simulink model "LGS_allFaultsDeselected"  (R2019b)
settings: Solver=FixedStepDiscrete  StartTime=0.0  StopTime=45.0  FixedStep=0.1  RelTol=1e-3
model workspace (MAT data in the model file):
  fipData : object (value not decoded)
  fipName : object (value not decoded)
  stepSize = 0.1
libraries: LibFaultInjectionControls x190, commrandsrc3 x70, simulink x3, LibFailureCondition x1
(part 3 of 41)

== system LGS_allFaultsDeselected/Doors/EV open doors ==
  In1 : Inport
  In2 : Inport  Port=2
  EV open doors : Stateflow chart  TreatAsAtomicUnit=on
  EV open doors FIP : Subsystem  Commented=on  mask(FailureInjectionPoint){}
      mask help: FailureInjectionPoint
      mask init: same as LGS_allFaultsDeselected/Analogical switch and general electro-valve and pressure sensor/Analogical switch/Analog Switch FIP
      settings: OpenFcn=|
      | open_system(gcb,'mask');
      | 
      | treeValues = FailureInjectionPointHelper.getAllFmAndParamsAsTreeString(gcb);
      | mo = Simulink.Mask.get(gcb);
      | dc = mo.getDialogControl('GbFmInfo');
      | treeView = dc.getDialogControl('TreeViewFM');
      | treeView.TreeItems = {};
      | treeView.TreeItems = treeValues;
      mask Help: FailureInjectionPoint
      mask DialogControl Control7 Prompt: Containing Failure Modes
      mask DialogControl BtnMoveUp Prompt: Move up
      mask DialogControl BtnMoveUp Callback:
      | %Get name of the failure mode block
      | mo = Simulink.Mask.get(gcb);
      | dc = mo.getDialogControl('GbFmInfo');
      | treeView = dc.getDialogControl('TreeViewFM');
      | try
      |     a = treeView.getSelectedItems();
      |     p = split(a, '/'); %name of failure mode block is p{1}
      | catch
      |     return;
      | end
      | 
      | %Save port handles
      | lh = get_param([gcb,'/',p{1}],'LineHandles');
      | ph = get_param([gcb,'/',p{1}],'PortHandles');
      | this_in = ph.Inport(1);
      | this_out = ph.Outport(1);
      | 
      | last_block = get_param(lh.Inport(1),'SrcBlockHandle');
      | last_block_type = get_param(last_block,'BlockType');
      | if strcmp(last_block_type,'Inport')
      |     return;
      | end
      | lb_lh = get_param(last_block,'LineHandles');
      | 
      | last_out = get_param(lh.Inport(1),'SrcPortHandle');
      | last_in = get_param(lb_lh.Inport(1),'DstPortHandle');
      | next_to_last_out = get_param(lb_lh.Inport(1),'SrcPortHandle');
      | next_in = get_param(lh.Outport(1),'DstPortHandle');
      | 
      | %Delete connecting lines
      | delete_line(lh.Inport(1));
      | delete_line(lh.Outport(1));
      | delete_line(lb_lh.Inport(1));
      | 
      | % Generate new lines
      | add_line(gcb, last_out, next_in, 'autorouting', 'smart');
      | add_line(gcb, this_out, last_in, 'autorouting', 'smart');
      | add_line(gcb, next_to_last_out, this_in, 'autorouting', 'smart');
      | 
      | %Rearrange system
      | Simulink.BlockDiagram.arrangeSystem(gcb);
      | 
      | %Refresh
      | treeValues = FailureInjectionPointHelper.getAllFmAndParamsAsTreeString(gcb);
      | mo = Simulink.Mask.get(gcb);
      | dc = mo.getDialogControl('GbFmInfo');
      | treeView = dc.getDialogControl('TreeViewFM');
      | treeView.TreeItems = {};
      | treeView.TreeItems = treeValues;
      mask DialogControl BtnMoveDown Prompt: Move down
      mask DialogControl BtnMoveDown Callback:
      | %Get name of the failure mode block
      | mo = Simulink.Mask.get(gcb);
      | dc = mo.getDialogControl('GbFmInfo');
      | treeView = dc.getDialogControl('TreeViewFM');
      | try
      |     a = treeView.getSelectedItems();
      |     p = split(a, '/'); %name of failure mode block is p{1}
      | catch
      |     return;
      | end
      | 
      | %Save port handles
      | lh = get_param([gcb,'/',p{1}],'LineHandles');
      | ph = get_param([gcb,'/',p{1}],'PortHandles');
      | this_in = ph.Inport(1);
      | this_out = ph.Outport(1);
      | 
      | next_block = get_param(lh.Outport(1),'DstBlockHandle');
      | next_block_type = get_param(next_block,'BlockType');
      | if strcmp(next_block_type,'Outport')
      |     return;
      | end
      | nb_lh = get_param(next_block,'LineHandles');
      | 
      | last_out = get_param(lh.Inport(1),'SrcPortHandle');
      | next_out = get_param(nb_lh.Outport(1),'SrcPortHandle');
      | next_but_one_in = get_param(nb_lh.Outport(1),'DstPortHandle');
      | next_in = get_param(lh.Outport(1),'DstPortHandle');
      | 
      | %Delete connecting lines
      | delete_line(lh.Inport(1));
      | delete_line(lh.Outport(1));
      | delete_line(nb_lh.Outport(1));
      | 
      | % Generate new lines
      | add_line(gcb, last_out, next_in, 'autorouting', 'smart');
      | add_line(gcb, next_out, this_in, 'autorouting', 'smart');
      | add_line(gcb, this_out, next_but_one_in, 'autorouting', 'smart');
      | 
      | %Rearrange system
      | Simulink.BlockDiagram.arrangeSystem(gcb);
      | 
      | %Refresh
      | treeValues = FailureInjectionPointHelper.getAllFmAndParamsAsTreeString(gcb);
      | mo = Simulink.Mask.get(gcb);
      | dc = mo.getDialogControl('GbFmInfo');
      | treeView = dc.getDialogControl('TreeViewFM');
      | treeView.TreeItems = {};
      | treeView.TreeItems = treeValues;
      mask DialogControl TreeViewFM Prompt: Failure Mode Information
      mask DialogControl BtnOpen Prompt: Open FIP
      mask DialogControl BtnOpen Callback: open_system(gcb,'force');
      mask DialogControl BtnNew Prompt: New
      mask DialogControl BtnNew Callback:
      | dialog_fipManager_single(gcb, '');
      | 
      | %Enable move, edit, delete buttons
      | mo = Simulink.Mask.get(gcb);
      | mo.getDialogControl('BtnMoveUp').Enabled = 'on';
      | mo.getDialogControl('BtnMoveDown').Enabled = 'on';
      | mo.getDialogControl('BtnEdit').Enabled = 'on';
      | mo.getDialogControl('BtnDelete').Enabled = 'on';
      mask DialogControl BtnEdit Prompt: Edit
      mask DialogControl BtnEdit Callback:
      | mo = Simulink.Mask.get(gcb);
      | dc = mo.getDialogControl('GbFmInfo');
      | treeView = dc.getDialogControl('TreeViewFM');
      | try
      |     a = treeView.getSelectedItems();
      |     p = split(a, '/');
      | catch
      |     return;
      | end
      | dialog_fipManager_single(gcb, p{1});
      mask DialogControl BtnDelete Prompt: Delete
      mask DialogControl BtnDelete Callback:
      | %Get name of the failure mode block
      | mo = Simulink.Mask.get(gcb);
      | dc = mo.getDialogControl('GbFmInfo');
      | treeView = dc.getDialogControl('TreeViewFM');
      | try
      |     a = treeView.getSelectedItems();
      |     p = split(a, '/'); %name of failure mode block is p{1}
      | catch
      |     return;
      | end
      | 
      | %Save outport handle of the last and inport handle of the next block
      | lh = get_param([gcb,'/',p{1}],'LineHandles');
      | last_out = get_param(lh.Inport(1),'SrcPortHandle');
      | next_in = get_param(lh.Outport(1),'DstPortHandle');
      | 
      | %Delete connecting lines and failure mode block
      | delete_line(lh.Inport(1));
      | delete_line(lh.Outport(1));
      | fm_handle = get_param([gcb,'/',p{1}],'Handle');
      | delete_block(fm_handle);
      | 
      | % Generate new line from outport last to inport next
      | add_line(gcb, last_out, next_in, 'autorouting', 'smart');
      | 
      | %Rearrange system
      | Simulink.BlockDiagram.arrangeSystem(gcb);
      | 
      | %Disable move, edit, delete buttons in case all FMs are deleted
      | last_block = get_param(last_out,'Parent');
      | last_is_inport = strcmp(get_param(last_block,'BlockType'),'Inport');
      | next_block = get_param(next_in,'Parent');
      | next_is_outport = strcmp(get_param(next_block,'BlockType'),'Outport');
      | if (last_is_inport && next_is_outport)
      |     mo.getDialogControl('BtnMoveUp').Enabled = 'off';
      |     mo.getDialogControl('BtnMoveDown').Enabled = 'off';
      |     mo.getDialogControl('BtnEdit').Enabled = 'off';
      |     mo.getDialogControl('BtnDelete').Enabled = 'off';
      | end
      | 
      | %Refresh
      | treeValues = FailureInjectionPointHelper.getAllFmAndParamsAsTreeString(gcb);
      | mo = Simulink.Mask.get(gcb);
      | dc = mo.getDialogControl('GbFmInfo');
      | treeView = dc.getDialogControl('TreeViewFM');
      | treeView.TreeItems = {};
      | treeView.TreeItems = treeValues;
      mask DialogControl BtnRefresh Prompt: Refresh
      mask DialogControl BtnRefresh Callback:
      | set_param(gcb,'LinkStatus','none');
      | 
      | treeValues = FailureInjectionPointHelper.getAllFmAndParamsAsTreeString(gcb);
      | mo = Simulink.Mask.get(gcb);
      | dc = mo.getDialogControl('GbFmInfo');
      | treeView = dc.getDialogControl('TreeViewFM');
      | treeView.TreeItems = {};
      | treeView.TreeItems = treeValues;
      mask Display: image('icons/failure_injection_point.png','center')
  Memory1 : Memory  InheritSampleTime=on
  Trigger FIP : LibFaultInjectionControls/Trigger FIP  Active=off  MaintenanceTask=1  RiskTime=1  FailureRate=1.0E-3  isDSF=off  DSFjson=JSON
      settings: SourceProductName=Fault Injection Controls
  Out1 : Outport
  wires:
  Memory1/1 -> EV open doors/1(signal_in)
  In1/1 -> Memory1/1
  In2/1 -> EV open doors/2(EVOpenDoorsPresure_in)
  Trigger FIP/1 -> EV open doors/3(fail)
  EV open doors/1(EVOpenDoorsPresure_out) -> Out1/1

== system LGS_allFaultsDeselected/Doors/front door zylinder ==
  note: [true, false]
  note: [true, false]
  presure open door : Inport  OutDataTypeStr=boolean
  presure close door : Inport  Port=2  OutDataTypeStr=boolean
  FD cylinder FIP : LibFaultInjectionControls/Trigger FIP  Active=off  MaintenanceTask=1  RiskTime=1  FailureRate=1.0E-3  isDSF=off  DSFjson=JSON
      settings: SourceProductName=Fault Injection Controls
  door cylinder : Stateflow chart  TreatAsAtomicUnit=on
  sensor locked closed : Subsystem
  sensor open : Subsystem
  sensor locked closed output : Outport
  sensor open output : Outport  Port=2
  door locked closed : Outport  Port=3
  wires:
  sensor open/1(sensor output) -> sensor open output/1
  sensor locked closed/1(sensor output) -> sensor locked closed output/1
  door cylinder/1(doorZylinderLockedClosed) -> door locked closed/1, sensor locked closed/1(sensor input)
  door cylinder/2(doorZylinderOpen) -> sensor open/1(sensor input)
  presure open door/1 -> door cylinder/1(presureOpenDoor)
  presure close door/1 -> door cylinder/2(presureCloseDoor)
  FD cylinder FIP/1 -> door cylinder/3(fail)

== system LGS_allFaultsDeselected/Doors/left door zylinder ==
  note: [true, false]
  note: [true, false]
  presure open door : Inport  OutDataTypeStr=boolean
  presure close door : Inport  Port=2  OutDataTypeStr=boolean
  LD cylinder FIP : LibFaultInjectionControls/Trigger FIP  Active=off  MaintenanceTask=1  RiskTime=1  FailureRate=1.0E-3  isDSF=off  DSFjson=JSON
      settings: SourceProductName=Fault Injection Controls
  door zylinder : Stateflow chart  TreatAsAtomicUnit=on
  sensor locked closed : Subsystem
  sensor open : Subsystem
  sensor locked closed output : Outport
  sensor open output : Outport  Port=2
  door locked closed : Outport  Port=3
  wires:
  LD cylinder FIP/1 -> door zylinder/3(fail)
  sensor open/1(sensor output) -> sensor open output/1
  sensor locked closed/1(sensor output) -> sensor locked closed output/1
  door zylinder/2(doorZylinderOpen) -> sensor open/1(sensor input)
  presure open door/1 -> door zylinder/1(presureOpenDoor)
  presure close door/1 -> door zylinder/2(presureCloseDoor)
  door zylinder/1(doorZylinderLockedClosed) -> door locked closed/1, sensor locked closed/1(sensor input)

== system LGS_allFaultsDeselected/Doors/right door zylinder ==
  note: [true, false]
  note: [true, false]
  presure open door : Inport  OutDataTypeStr=boolean
  presure close door : Inport  Port=2  OutDataTypeStr=boolean
  RD cylinder FIP : LibFaultInjectionControls/Trigger FIP  Active=off  MaintenanceTask=1  RiskTime=1  FailureRate=1.0E-3  isDSF=off  DSFjson=JSON
      settings: SourceProductName=Fault Injection Controls
  door zylinder : Stateflow chart  TreatAsAtomicUnit=on
  sensor locked closed : Subsystem
  sensor open : Subsystem
  sensor locked closed output : Outport
  sensor open output : Outport  Port=2
  door locked closed : Outport  Port=3
  wires:
  RD cylinder FIP/1 -> door zylinder/3(fail)
  sensor open/1(sensor output) -> sensor open output/1
  sensor locked closed/1(sensor output) -> sensor locked closed output/1
  door zylinder/2(doorZylinderOpen) -> sensor open/1(sensor input)
  presure open door/1 -> door zylinder/1(presureOpenDoor)
  presure close door/1 -> door zylinder/2(presureCloseDoor)
  door zylinder/1(doorZylinderLockedClosed) -> door locked closed/1, sensor locked closed/1(sensor input)

== system LGS_allFaultsDeselected/FailureConditionObserver/FC1 ==
  Retraction Valve : Inport
  Extension Valve : Inport  Port=2
  ActualSystemCondition : Subsystem  AncestorBlock=LibFailureCondition/ActualSystemCondition  mask(ActualSystemCondition){}
      mask help: ActualSystemCondition
      mask Help: ActualSystemCondition
  FC1 : Terminator  mask(DiveObserver){}
      mask help: DiveObserver
      settings: AncestorBlock=LibFailureCondition/DiveObserver
      mask Help: DiveObserver
      mask Display: image('icons/observer.png','center')
  FC_FC1_output : Subsystem  AncestorBlock=LibFailureCondition/ExpectedSystemBehavior  mask(ExpectedSystemBehavior){}
      mask help: ExpectedSystemBehavior
      mask Help: ExpectedSystemBehavior
  wires:
  ActualSystemCondition/1("Activate Observer ") -> FC_FC1_output/1(ActivateObserver)
  FC_FC1_output/1(ConditionState) -> FC1/1
  Retraction Valve/1 -> FC_FC1_output/2(Retraction Valve)
  Extension Valve/1 -> FC_FC1_output/3(Extension Valve)

== system LGS_allFaultsDeselected/FailureConditionObserver/FC2 ==
  Red LED : Inport
  FG locked extended : Inport  Port=2
  "LG locked extended " : Inport  Port=3
  RG locked extended : Inport  Port=4
  FD locked closed : Inport  Port=5
  LD locked closed : Inport  Port=6
  RD locked closed : Inport  Port=7
  Command Handle : Inport  Port=8
  ActualSystemCondition : Subsystem  AncestorBlock=LibFailureCondition/ActualSystemCondition  mask(ActualSystemCondition){}
      mask help: ActualSystemCondition
      mask Help: ActualSystemCondition
  FC2 : Terminator  mask(DiveObserver){}
      mask help: DiveObserver
      settings: AncestorBlock=LibFailureCondition/DiveObserver
      mask Help: DiveObserver
      mask Display: image('icons/observer.png','center')
  FC_FC2_output : Subsystem  AncestorBlock=LibFailureCondition/ExpectedSystemBehavior  mask(ExpectedSystemBehavior){}
      mask help: ExpectedSystemBehavior
      mask Help: ExpectedSystemBehavior
  wires:
  FC_FC2_output/1(ConditionState) -> FC2/1
  ActualSystemCondition/1("Activate Observer ") -> FC_FC2_output/1(ActivateObserver)
  Red LED/1 -> FC_FC2_output/9(Red LED)
  FG locked extended/1 -> FC_FC2_output/3(FG locked down)
  RG locked extended/1 -> FC_FC2_output/4(RG locked down)
  RD locked closed/1 -> FC_FC2_output/7(RD locked closed)
  FD locked closed/1 -> FC_FC2_output/6(FD locked closed)
  LD locked closed/1 -> FC_FC2_output/8(LD locked closed)
  Command Handle/1 -> FC_FC2_output/2(Command Handle)
  "LG locked extended "/1 -> FC_FC2_output/5(LG locked down)

== system LGS_allFaultsDeselected/FailureConditionObserver/FC3 ==
  Green LED : Inport
  Orange LED : Inport  Port=2
  Red LED : Inport  Port=3
  FG locked extended : Inport  Port=4
  LG locked extended : Inport  Port=5
  RG locked extended : Inport  Port=6
  FD locked closed : Inport  Port=7
  LD locked closed : Inport  Port=8
  RD locked closed : Inport  Port=9
  ActualSystemCondition : Subsystem  AncestorBlock=LibFailureCondition/ActualSystemCondition  mask(ActualSystemCondition){}
      mask help: ActualSystemCondition
      mask Help: ActualSystemCondition
  FC3 : LibFailureCondition/DiveObserver
      settings: SourceProductName=Failure Condition
  FC_FC3_output : Subsystem  AncestorBlock=LibFailureCondition/ExpectedSystemBehavior  mask(ExpectedSystemBehavior){}
      mask help: ExpectedSystemBehavior
      mask Help: ExpectedSystemBehavior
  wires:
  FC_FC3_output/1(ConditionState) -> FC3/1
  ActualSystemCondition/1("Activate Observer ") -> FC_FC3_output/1(ActivateObserver)
  Green LED/1 -> ActualSystemCondition/1(Green LED)
  Orange LED/1 -> ActualSystemCondition/2(Orange LED)
  Red LED/1 -> ActualSystemCondition/3(Red LED)
  FG locked extended/1 -> FC_FC3_output/2(FG locked down)
  LG locked extended/1 -> FC_FC3_output/4(LG locked down)
  RG locked extended/1 -> FC_FC3_output/3(RG locked down)
  FD locked closed/1 -> FC_FC3_output/5(FD locked closed1)
  LD locked closed/1 -> FC_FC3_output/7(LD locked closed1)
  RD locked closed/1 -> FC_FC3_output/6(RD locked closed1)

== system LGS_allFaultsDeselected/Gears/EV extend gear ==
  In1 : Inport
  In2 : Inport  Port=2
  EV extend gear : Stateflow chart  TreatAsAtomicUnit=on
  EV extend gear FIP : Subsystem  Commented=on  mask(FailureInjectionPoint){}
      mask help: FailureInjectionPoint
      mask init: same as LGS_allFaultsDeselected/Analogical switch and general electro-valve and pressure sensor/Analogical switch/Analog Switch FIP
      settings: OpenFcn=|
      | open_system(gcb,'mask');
      | 
      | treeValues = FailureInjectionPointHelper.getAllFmAndParamsAsTreeString(gcb);
      | mo = Simulink.Mask.get(gcb);
      | dc = mo.getDialogControl('GbFmInfo');
      | treeView = dc.getDialogControl('TreeViewFM');
      | treeView.TreeItems = {};
      | treeView.TreeItems = treeValues;
      mask Help: FailureInjectionPoint
      mask DialogControl Control7 Prompt: Containing Failure Modes
      mask DialogControl BtnMoveUp Prompt: Move up
      mask DialogControl BtnMoveUp Callback:
      | %Get name of the failure mode block
      | mo = Simulink.Mask.get(gcb);
      | dc = mo.getDialogControl('GbFmInfo');
      | treeView = dc.getDialogControl('TreeViewFM');
      | try
      |     a = treeView.getSelectedItems();
      |     p = split(a, '/'); %name of failure mode block is p{1}
      | catch
      |     return;
      | end
      | 
      | %Save port handles
      | lh = get_param([gcb,'/',p{1}],'LineHandles');
      | ph = get_param([gcb,'/',p{1}],'PortHandles');
      | this_in = ph.Inport(1);
      | this_out = ph.Outport(1);
      | 
      | last_block = get_param(lh.Inport(1),'SrcBlockHandle');
      | last_block_type = get_param(last_block,'BlockType');
      | if strcmp(last_block_type,'Inport')
      |     return;
      | end
      | lb_lh = get_param(last_block,'LineHandles');
      | 
      | last_out = get_param(lh.Inport(1),'SrcPortHandle');
      | last_in = get_param(lb_lh.Inport(1),'DstPortHandle');
      | next_to_last_out = get_param(lb_lh.Inport(1),'SrcPortHandle');
      | next_in = get_param(lh.Outport(1),'DstPortHandle');
      | 
      | %Delete connecting lines
      | delete_line(lh.Inport(1));
      | delete_line(lh.Outport(1));
      | delete_line(lb_lh.Inport(1));
      | 
      | % Generate new lines
      | add_line(gcb, last_out, next_in, 'autorouting', 'smart');
      | add_line(gcb, this_out, last_in, 'autorouting', 'smart');
      | add_line(gcb, next_to_last_out, this_in, 'autorouting', 'smart');
      | 
      | %Rearrange system
      | Simulink.BlockDiagram.arrangeSystem(gcb);
      | 
      | %Refresh
      | treeValues = FailureInjectionPointHelper.getAllFmAndParamsAsTreeString(gcb);
      | mo = Simulink.Mask.get(gcb);
      | dc = mo.getDialogControl('GbFmInfo');
      | treeView = dc.getDialogControl('TreeViewFM');
      | treeView.TreeItems = {};
      | treeView.TreeItems = treeValues;
      mask DialogControl BtnMoveDown Prompt: Move down
      mask DialogControl BtnMoveDown Callback:
      | %Get name of the failure mode block
      | mo = Simulink.Mask.get(gcb);
      | dc = mo.getDialogControl('GbFmInfo');
      | treeView = dc.getDialogControl('TreeViewFM');
      | try
      |     a = treeView.getSelectedItems();
      |     p = split(a, '/'); %name of failure mode block is p{1}
      | catch
      |     return;
      | end
      | 
      | %Save port handles
      | lh = get_param([gcb,'/',p{1}],'LineHandles');
      | ph = get_param([gcb,'/',p{1}],'PortHandles');
      | this_in = ph.Inport(1);
      | this_out = ph.Outport(1);
      | 
      | next_block = get_param(lh.Outport(1),'DstBlockHandle');
      | next_block_type = get_param(next_block,'BlockType');
      | if strcmp(next_block_type,'Outport')
      |     return;
      | end
      | nb_lh = get_param(next_block,'LineHandles');
      | 
      | last_out = get_param(lh.Inport(1),'SrcPortHandle');
      | next_out = get_param(nb_lh.Outport(1),'SrcPortHandle');
      | next_but_one_in = get_param(nb_lh.Outport(1),'DstPortHandle');
      | next_in = get_param(lh.Outport(1),'DstPortHandle');
      | 
      | %Delete connecting lines
      | delete_line(lh.Inport(1));
      | delete_line(lh.Outport(1));
      | delete_line(nb_lh.Outport(1));
      | 
      | % Generate new lines
      | add_line(gcb, last_out, next_in, 'autorouting', 'smart');
      | add_line(gcb, next_out, this_in, 'autorouting', 'smart');
      | add_line(gcb, this_out, next_but_one_in, 'autorouting', 'smart');
      | 
      | %Rearrange system
      | Simulink.BlockDiagram.arrangeSystem(gcb);
      | 
      | %Refresh
      | treeValues = FailureInjectionPointHelper.getAllFmAndParamsAsTreeString(gcb);
      | mo = Simulink.Mask.get(gcb);
      | dc = mo.getDialogControl('GbFmInfo');
      | treeView = dc.getDialogControl('TreeViewFM');
      | treeView.TreeItems = {};
      | treeView.TreeItems = treeValues;
      mask DialogControl TreeViewFM Prompt: Failure Mode Information
      mask DialogControl BtnOpen Prompt: Open FIP
      mask DialogControl BtnOpen Callback: open_system(gcb,'force');
      mask DialogControl BtnNew Prompt: New
      mask DialogControl BtnNew Callback:
      | dialog_fipManager_single(gcb, '');
      | 
      | %Enable move, edit, delete buttons
      | mo = Simulink.Mask.get(gcb);
      | mo.getDialogControl('BtnMoveUp').Enabled = 'on';
      | mo.getDialogControl('BtnMoveDown').Enabled = 'on';
      | mo.getDialogControl('BtnEdit').Enabled = 'on';
      | mo.getDialogControl('BtnDelete').Enabled = 'on';
      mask DialogControl BtnEdit Prompt: Edit
      mask DialogControl BtnEdit Callback:
      | mo = Simulink.Mask.get(gcb);
      | dc = mo.getDialogControl('GbFmInfo');
      | treeView = dc.getDialogControl('TreeViewFM');
      | try
      |     a = treeView.getSelectedItems();
      |     p = split(a, '/');
      | catch
      |     return;
      | end
      | dialog_fipManager_single(gcb, p{1});
      mask DialogControl BtnDelete Prompt: Delete
      mask DialogControl BtnDelete Callback:
      | %Get name of the failure mode block
      | mo = Simulink.Mask.get(gcb);
      | dc = mo.getDialogControl('GbFmInfo');
      | treeView = dc.getDialogControl('TreeViewFM');
      | try
      |     a = treeView.getSelectedItems();
      |     p = split(a, '/'); %name of failure mode block is p{1}
      | catch
      |     return;
      | end
      | 
      | %Save outport handle of the last and inport handle of the next block
      | lh = get_param([gcb,'/',p{1}],'LineHandles');
      | last_out = get_param(lh.Inport(1),'SrcPortHandle');
      | next_in = get_param(lh.Outport(1),'DstPortHandle');
      | 
      | %Delete connecting lines and failure mode block
      | delete_line(lh.Inport(1));
      | delete_line(lh.Outport(1));
      | fm_handle = get_param([gcb,'/',p{1}],'Handle');
      | delete_block(fm_handle);
      | 
      | % Generate new line from outport last to inport next
      | add_line(gcb, last_out, next_in, 'autorouting', 'smart');
      | 
      | %Rearrange system
      | Simulink.BlockDiagram.arrangeSystem(gcb);
      | 
      | %Disable move, edit, delete buttons in case all FMs are deleted
      | last_block = get_param(last_out,'Parent');
      | last_is_inport = strcmp(get_param(last_block,'BlockType'),'Inport');
      | next_block = get_param(next_in,'Parent');
      | next_is_outport = strcmp(get_param(next_block,'BlockType'),'Outport');
      | if (last_is_inport && next_is_outport)
      |     mo.getDialogControl('BtnMoveUp').Enabled = 'off';
      |     mo.getDialogControl('BtnMoveDown').Enabled = 'off';
      |     mo.getDialogControl('BtnEdit').Enabled = 'off';
      |     mo.getDialogControl('BtnDelete').Enabled = 'off';
      | end
      | 
      | %Refresh
      | treeValues = FailureInjectionPointHelper.getAllFmAndParamsAsTreeString(gcb);
      | mo = Simulink.Mask.get(gcb);
      | dc = mo.getDialogControl('GbFmInfo');
      | treeView = dc.getDialogControl('TreeViewFM');
      | treeView.TreeItems = {};
      | treeView.TreeItems = treeValues;
      mask DialogControl BtnRefresh Prompt: Refresh
      mask DialogControl BtnRefresh Callback:
      | set_param(gcb,'LinkStatus','none');
      | 
      | treeValues = FailureInjectionPointHelper.getAllFmAndParamsAsTreeString(gcb);
      | mo = Simulink.Mask.get(gcb);
      | dc = mo.getDialogControl('GbFmInfo');
      | treeView = dc.getDialogControl('TreeViewFM');
      | treeView.TreeItems = {};
      | treeView.TreeItems = treeValues;
      mask Display: image('icons/failure_injection_point.png','center')
  Memory : Memory  InheritSampleTime=on
  Trigger FIP : LibFaultInjectionControls/Trigger FIP  Active=off  MaintenanceTask=1  RiskTime=1  FailureRate=1.0E-3  isDSF=off  DSFjson=JSON
      settings: SourceProductName=Fault Injection Controls
  Out1 : Outport
  wires:
  Memory/1 -> EV extend gear/1(signal_in)
  In1/1 -> Memory/1
  In2/1 -> EV extend gear/2(EVExtendGearPresure_in)
  Trigger FIP/1 -> EV extend gear/3(fail)
  EV extend gear/1(EVExtendGearPresure_out) -> Out1/1

== system LGS_allFaultsDeselected/Gears/EV retract gear ==
  In1 : Inport
  In2 : Inport  Port=2
  EV retract gear : Stateflow chart  TreatAsAtomicUnit=on
  EV retract gear FIP : Subsystem  Commented=on  mask(FailureInjectionPoint){}
      mask help: FailureInjectionPoint
      mask init: same as LGS_allFaultsDeselected/Analogical switch and general electro-valve and pressure sensor/Analogical switch/Analog Switch FIP
      settings: OpenFcn=|
      | open_system(gcb,'mask');
      | 
      | treeValues = FailureInjectionPointHelper.getAllFmAndParamsAsTreeString(gcb);
      | mo = Simulink.Mask.get(gcb);
      | dc = mo.getDialogControl('GbFmInfo');
      | treeView = dc.getDialogControl('TreeViewFM');
      | treeView.TreeItems = {};
      | treeView.TreeItems = treeValues;
      mask Help: FailureInjectionPoint
      mask DialogControl Control7 Prompt: Containing Failure Modes
      mask DialogControl BtnMoveUp Prompt: Move up
      mask DialogControl BtnMoveUp Callback:
      | %Get name of the failure mode block
      | mo = Simulink.Mask.get(gcb);
      | dc = mo.getDialogControl('GbFmInfo');
      | treeView = dc.getDialogControl('TreeViewFM');
      | try
      |     a = treeView.getSelectedItems();
      |     p = split(a, '/'); %name of failure mode block is p{1}
      | catch
      |     return;
      | end
      | 
      | %Save port handles
      | lh = get_param([gcb,'/',p{1}],'LineHandles');
      | ph = get_param([gcb,'/',p{1}],'PortHandles');
      | this_in = ph.Inport(1);
      | this_out = ph.Outport(1);
      | 
      | last_block = get_param(lh.Inport(1),'SrcBlockHandle');
      | last_block_type = get_param(last_block,'BlockType');
      | if strcmp(last_block_type,'Inport')
      |     return;
      | end
      | lb_lh = get_param(last_block,'LineHandles');
      | 
      | last_out = get_param(lh.Inport(1),'SrcPortHandle');
      | last_in = get_param(lb_lh.Inport(1),'DstPortHandle');
      | next_to_last_out = get_param(lb_lh.Inport(1),'SrcPortHandle');
      | next_in = get_param(lh.Outport(1),'DstPortHandle');
      | 
      | %Delete connecting lines
      | delete_line(lh.Inport(1));
      | delete_line(lh.Outport(1));
      | delete_line(lb_lh.Inport(1));
      | 
      | % Generate new lines
      | add_line(gcb, last_out, next_in, 'autorouting', 'smart');
      | add_line(gcb, this_out, last_in, 'autorouting', 'smart');
      | add_line(gcb, next_to_last_out, this_in, 'autorouting', 'smart');
      | 
      | %Rearrange system
      | Simulink.BlockDiagram.arrangeSystem(gcb);
      | 
      | %Refresh
      | treeValues = FailureInjectionPointHelper.getAllFmAndParamsAsTreeString(gcb);
      | mo = Simulink.Mask.get(gcb);
      | dc = mo.getDialogControl('GbFmInfo');
      | treeView = dc.getDialogControl('TreeViewFM');
      | treeView.TreeItems = {};
      | treeView.TreeItems = treeValues;
      mask DialogControl BtnMoveDown Prompt: Move down
      mask DialogControl BtnMoveDown Callback:
      | %Get name of the failure mode block
      | mo = Simulink.Mask.get(gcb);
      | dc = mo.getDialogControl('GbFmInfo');
      | treeView = dc.getDialogControl('TreeViewFM');
      | try
      |     a = treeView.getSelectedItems();
      |     p = split(a, '/'); %name of failure mode block is p{1}
      | catch
      |     return;
      | end
      | 
      | %Save port handles
      | lh = get_param([gcb,'/',p{1}],'LineHandles');
      | ph = get_param([gcb,'/',p{1}],'PortHandles');
      | this_in = ph.Inport(1);
      | this_out = ph.Outport(1);
      | 
      | next_block = get_param(lh.Outport(1),'DstBlockHandle');
      | next_block_type = get_param(next_block,'BlockType');
      | if strcmp(next_block_type,'Outport')
      |     return;
      | end
      | nb_lh = get_param(next_block,'LineHandles');
      | 
      | last_out = get_param(lh.Inport(1),'SrcPortHandle');
      | next_out = get_param(nb_lh.Outport(1),'SrcPortHandle');
      | next_but_one_in = get_param(nb_lh.Outport(1),'DstPortHandle');
      | next_in = get_param(lh.Outport(1),'DstPortHandle');
      | 
      | %Delete connecting lines
      | delete_line(lh.Inport(1));
      | delete_line(lh.Outport(1));
      | delete_line(nb_lh.Outport(1));
      | 
      | % Generate new lines
      | add_line(gcb, last_out, next_in, 'autorouting', 'smart');
      | add_line(gcb, next_out, this_in, 'autorouting', 'smart');
      | add_line(gcb, this_out, next_but_one_in, 'autorouting', 'smart');
      | 
      | %Rearrange system
      | Simulink.BlockDiagram.arrangeSystem(gcb);
      | 
      | %Refresh
      | treeValues = FailureInjectionPointHelper.getAllFmAndParamsAsTreeString(gcb);
      | mo = Simulink.Mask.get(gcb);
      | dc = mo.getDialogControl('GbFmInfo');
      | treeView = dc.getDialogControl('TreeViewFM');
      | treeView.TreeItems = {};
      | treeView.TreeItems = treeValues;
      mask DialogControl TreeViewFM Prompt: Failure Mode Information
      mask DialogControl BtnOpen Prompt: Open FIP
      mask DialogControl BtnOpen Callback: open_system(gcb,'force');
      mask DialogControl BtnNew Prompt: New
      mask DialogControl BtnNew Callback:
      | dialog_fipManager_single(gcb, '');
      | 
      | %Enable move, edit, delete buttons
      | mo = Simulink.Mask.get(gcb);
      | mo.getDialogControl('BtnMoveUp').Enabled = 'on';
      | mo.getDialogControl('BtnMoveDown').Enabled = 'on';
      | mo.getDialogControl('BtnEdit').Enabled = 'on';
      | mo.getDialogControl('BtnDelete').Enabled = 'on';
      mask DialogControl BtnEdit Prompt: Edit
      mask DialogControl BtnEdit Callback:
      | mo = Simulink.Mask.get(gcb);
      | dc = mo.getDialogControl('GbFmInfo');
      | treeView = dc.getDialogControl('TreeViewFM');
      | try
      |     a = treeView.getSelectedItems();
      |     p = split(a, '/');
      | catch
      |     return;
      | end
      | dialog_fipManager_single(gcb, p{1});
      mask DialogControl BtnDelete Prompt: Delete
      mask DialogControl BtnDelete Callback:
      | %Get name of the failure mode block
      | mo = Simulink.Mask.get(gcb);
      | dc = mo.getDialogControl('GbFmInfo');
      | treeView = dc.getDialogControl('TreeViewFM');
      | try
      |     a = treeView.getSelectedItems();
      |     p = split(a, '/'); %name of failure mode block is p{1}
      | catch
      |     return;
      | end
      | 
      | %Save outport handle of the last and inport handle of the next block
      | lh = get_param([gcb,'/',p{1}],'LineHandles');
      | last_out = get_param(lh.Inport(1),'SrcPortHandle');
      | next_in = get_param(lh.Outport(1),'DstPortHandle');
      | 
      | %Delete connecting lines and failure mode block
      | delete_line(lh.Inport(1));
      | delete_line(lh.Outport(1));
      | fm_handle = get_param([gcb,'/',p{1}],'Handle');
      | delete_block(fm_handle);
      | 
      | % Generate new line from outport last to inport next
      | add_line(gcb, last_out, next_in, 'autorouting', 'smart');
      | 
      | %Rearrange system
      | Simulink.BlockDiagram.arrangeSystem(gcb);
      | 
      | %Disable move, edit, delete buttons in case all FMs are deleted
      | last_block = get_param(last_out,'Parent');
      | last_is_inport = strcmp(get_param(last_block,'BlockType'),'Inport');
      | next_block = get_param(next_in,'Parent');
      | next_is_outport = strcmp(get_param(next_block,'BlockType'),'Outport');
      | if (last_is_inport && next_is_outport)
      |     mo.getDialogControl('BtnMoveUp').Enabled = 'off';
      |     mo.getDialogControl('BtnMoveDown').Enabled = 'off';
      |     mo.getDialogControl('BtnEdit').Enabled = 'off';
      |     mo.getDialogControl('BtnDelete').Enabled = 'off';
      | end
      | 
      | %Refresh
      | treeValues = FailureInjectionPointHelper.getAllFmAndParamsAsTreeString(gcb);
      | mo = Simulink.Mask.get(gcb);
      | dc = mo.getDialogControl('GbFmInfo');
      | treeView = dc.getDialogControl('TreeViewFM');
      | treeView.TreeItems = {};
      | treeView.TreeItems = treeValues;
      mask DialogControl BtnRefresh Prompt: Refresh
      mask DialogControl BtnRefresh Callback:
      | set_param(gcb,'LinkStatus','none');
      | 
      | treeValues = FailureInjectionPointHelper.getAllFmAndParamsAsTreeString(gcb);
      | mo = Simulink.Mask.get(gcb);
      | dc = mo.getDialogControl('GbFmInfo');
      | treeView = dc.getDialogControl('TreeViewFM');
      | treeView.TreeItems = {};
      | treeView.TreeItems = treeValues;
      mask Display: image('icons/failure_injection_point.png','center')
  Memory1 : Memory  InheritSampleTime=on
  Trigger FIP : LibFaultInjectionControls/Trigger FIP  Active=off  MaintenanceTask=1  RiskTime=1  FailureRate=1.0E-3  isDSF=off  DSFjson=JSON
      settings: SourceProductName=Fault Injection Controls
  Out1 : Outport
  wires:
  Memory1/1 -> EV retract gear/1(signal_in)
  In1/1 -> Memory1/1
  In2/1 -> EV retract gear/2(EVRetractGearPresure_in)
  Trigger FIP/1 -> EV retract gear/3(fail)
  EV retract gear/1(EVRetractGearPresure_out) -> Out1/1

== system LGS_allFaultsDeselected/Gears/FG shock absorber ==
  shock absorber in : Inport  OutDataTypeStr=boolean
  sensor shock absorber : Subsystem
  sensor shock absorber output : Outport
  wires:
  shock absorber in/1 -> sensor shock absorber/1(sensor input)
  sensor shock absorber/1(sensor output) -> sensor shock absorber output/1

== system LGS_allFaultsDeselected/Gears/LG shock absorber ==
  shock absorber in : Inport  OutDataTypeStr=boolean
  sensor shock absorber : Subsystem
  sensor shock absorber output : Outport
  wires:
  shock absorber in/1 -> sensor shock absorber/1(sensor input)
  sensor shock absorber/1(sensor output) -> sensor shock absorber output/1

== system LGS_allFaultsDeselected/Gears/RG shock absorber ==
  shock absorber in : Inport  OutDataTypeStr=boolean
  sensor shock absorber : Subsystem
  sensor shock absorber output : Outport
  wires:
  shock absorber in/1 -> sensor shock absorber/1(sensor input)
  sensor shock absorber/1(sensor output) -> sensor shock absorber output/1

== system LGS_allFaultsDeselected/Gears/front gear cylinder ==
  note: [true, false]
  note: [true, false]
  presure extend gear : Inport  OutDataTypeStr=boolean
  presure retract gear : Inport  Port=2  OutDataTypeStr=boolean
  initial handle state : Inport  Port=3
  FG cylinder FIP : LibFaultInjectionControls/Trigger FIP  Active=off  MaintenanceTask=1  RiskTime=1  FailureRate=1.0E-3  isDSF=off  DSFjson=JSON
      settings: SourceProductName=Fault Injection Controls
  gear zylinder : Stateflow chart  TreatAsAtomicUnit=on
  sensor locked extended : Subsystem
  sensor locked retracted : Subsystem
  sensor locked extended output : Outport
  sensor locked retracted output : Outport  Port=2
  gear locked extended : Outport  Port=3
  gear locked retracted : Outport  Port=4
  wires:
  FG cylinder FIP/1 -> gear zylinder/3(fail)
  presure retract gear/1 -> gear zylinder/2(presureRetractGear)
  presure extend gear/1 -> gear zylinder/1(presureExtendGear)
  gear zylinder/1(gearLockedExtended) -> gear locked extended/1, sensor locked extended/1(sensor input)
  sensor locked extended/1(sensor output) -> sensor locked extended output/1
  gear zylinder/2(gearLockedRetracted) -> gear locked retracted/1, sensor locked retracted/1(sensor input)
  sensor locked retracted/1(sensor output) -> sensor locked retracted output/1
  initial handle state/1 -> gear zylinder/4(initHandleState)

== system LGS_allFaultsDeselected/Gears/left gear cylinder ==
  note: [true, false]
  note: [true, false]
  presure extend gear : Inport  OutDataTypeStr=boolean
  presure retract gear : Inport  Port=2  OutDataTypeStr=boolean
  initial handle state : Inport  Port=3
  LG cylinder FIP : LibFaultInjectionControls/Trigger FIP  Active=off  MaintenanceTask=1  RiskTime=1  FailureRate=1.0E-3  isDSF=off  DSFjson=JSON
      settings: SourceProductName=Fault Injection Controls
  gear zylinder : Stateflow chart  TreatAsAtomicUnit=on
  sensor locked extended : Subsystem
  sensor locked retracted : Subsystem
  sensor locked extended output : Outport
  sensor locked retracted output : Outport  Port=2
  gear locked extended : Outport  Port=3
  gear locked retracted : Outport  Port=4
  wires:
  LG cylinder FIP/1 -> gear zylinder/3(fail)
  presure retract gear/1 -> gear zylinder/2(presureRetractGear)
  presure extend gear/1 -> gear zylinder/1(presureExtendGear)
  sensor locked extended/1(sensor output) -> sensor locked extended output/1
  sensor locked retracted/1(sensor output) -> sensor locked retracted output/1
  gear zylinder/1(gearLockedExtended) -> gear locked extended/1, sensor locked extended/1(sensor input)
  gear zylinder/2(gearLockedRetracted) -> gear locked retracted/1, sensor locked retracted/1(sensor input)
  initial handle state/1 -> gear zylinder/4(initHandleState)

== system LGS_allFaultsDeselected/Gears/right gear cylinder ==
  note: [true, false]
  note: [true, false]
  presure extend gear : Inport  OutDataTypeStr=boolean
  presure retract gear : Inport  Port=2  OutDataTypeStr=boolean
  initial handle state : Inport  Port=3
  RG cylinder FIP : LibFaultInjectionControls/Trigger FIP  Active=off  MaintenanceTask=1  RiskTime=1  FailureRate=1.0E-3  isDSF=off  DSFjson=JSON
      settings: SourceProductName=Fault Injection Controls
  gear zylinder : Stateflow chart  TreatAsAtomicUnit=on
  sensor locked extended : Subsystem
  sensor locked retracted : Subsystem
  sensor locked extended output : Outport
  sensor locked retracted output : Outport  Port=2
  gear locked extended : Outport  Port=3
  gear locked retracted : Outport  Port=4
  wires:
  RG cylinder FIP/1 -> gear zylinder/3(fail)
  presure retract gear/1 -> gear zylinder/2(presureRetractGear)
  presure extend gear/1 -> gear zylinder/1(presureExtendGear)
  sensor locked extended/1(sensor output) -> sensor locked extended output/1
  sensor locked retracted/1(sensor output) -> sensor locked retracted output/1
  gear zylinder/1(gearLockedExtended) -> gear locked extended/1, sensor locked extended/1(sensor input)
  gear zylinder/2(gearLockedRetracted) -> gear locked retracted/1, sensor locked retracted/1(sensor input)
  initial handle state/1 -> gear zylinder/4(initHandleState)

== system LGS_allFaultsDeselected/sensor up down handle/FIP1 ==
  In1 : Inport
  Handle sensor FIP1 : Subsystem  mask(FailureInjectionPoint){}
      mask help: FailureInjectionPoint
      mask init: same as LGS_allFaultsDeselected/Analogical switch and general electro-valve and pressure sensor/Analogical switch/Analog Switch FIP
      settings: OpenFcn=|
      | open_system(gcb,'mask');
      | 
      | treeValues = FailureInjectionPointHelper.getAllFmAndParamsAsTreeString(gcb);
      | mo = Simulink.Mask.get(gcb);
      | dc = mo.getDialogControl('GbFmInfo');
      | treeView = dc.getDialogControl('TreeViewFM');
      | treeView.TreeItems = {};
      | treeView.TreeItems = treeValues;
      mask Help: FailureInjectionPoint
      mask DialogControl Control7 Prompt: Containing Failure Modes
      mask DialogControl BtnMoveUp Prompt: Move up
      mask DialogControl BtnMoveUp Callback:
      | %Get name of the failure mode block
      | mo = Simulink.Mask.get(gcb);
      | dc = mo.getDialogControl('GbFmInfo');
      | treeView = dc.getDialogControl('TreeViewFM');
      | try
      |     a = treeView.getSelectedItems();
      |     p = split(a, '/'); %name of failure mode block is p{1}
      | catch
      |     return;
      | end
      | 
      | %Save port handles
      | lh = get_param([gcb,'/',p{1}],'LineHandles');
      | ph = get_param([gcb,'/',p{1}],'PortHandles');
      | this_in = ph.Inport(1);
      | this_out = ph.Outport(1);
      | 
      | last_block = get_param(lh.Inport(1),'SrcBlockHandle');
      | last_block_type = get_param(last_block,'BlockType');
      | if strcmp(last_block_type,'Inport')
      |     return;
      | end
      | lb_lh = get_param(last_block,'LineHandles');
      | 
      | last_out = get_param(lh.Inport(1),'SrcPortHandle');
      | last_in = get_param(lb_lh.Inport(1),'DstPortHandle');
      | next_to_last_out = get_param(lb_lh.Inport(1),'SrcPortHandle');
      | next_in = get_param(lh.Outport(1),'DstPortHandle');
      | 
      | %Delete connecting lines
      | delete_line(lh.Inport(1));
      | delete_line(lh.Outport(1));
      | delete_line(lb_lh.Inport(1));
      | 
      | % Generate new lines
      | add_line(gcb, last_out, next_in, 'autorouting', 'smart');
      | add_line(gcb, this_out, last_in, 'autorouting', 'smart');
      | add_line(gcb, next_to_last_out, this_in, 'autorouting', 'smart');
      | 
      | %Rearrange system
      | Simulink.BlockDiagram.arrangeSystem(gcb);
      | 
      | %Refresh
      | treeValues = FailureInjectionPointHelper.getAllFmAndParamsAsTreeString(gcb);
      | mo = Simulink.Mask.get(gcb);
      | dc = mo.getDialogControl('GbFmInfo');
      | treeView = dc.getDialogControl('TreeViewFM');
      | treeView.TreeItems = {};
      | treeView.TreeItems = treeValues;
      mask DialogControl BtnMoveDown Prompt: Move down
      mask DialogControl BtnMoveDown Callback:
      | %Get name of the failure mode block
      | mo = Simulink.Mask.get(gcb);
      | dc = mo.getDialogControl('GbFmInfo');
      | treeView = dc.getDialogControl('TreeViewFM');
      | try
      |     a = treeView.getSelectedItems();
      |     p = split(a, '/'); %name of failure mode block is p{1}
      | catch
      |     return;
      | end
      | 
      | %Save port handles
      | lh = get_param([gcb,'/',p{1}],'LineHandles');
      | ph = get_param([gcb,'/',p{1}],'PortHandles');
      | this_in = ph.Inport(1);
      | this_out = ph.Outport(1);
      | 
      | next_block = get_param(lh.Outport(1),'DstBlockHandle');
      | next_block_type = get_param(next_block,'BlockType');
      | if strcmp(next_block_type,'Outport')
      |     return;
      | end
      | nb_lh = get_param(next_block,'LineHandles');
      | 
      | last_out = get_param(lh.Inport(1),'SrcPortHandle');
      | next_out = get_param(nb_lh.Outport(1),'SrcPortHandle');
      | next_but_one_in = get_param(nb_lh.Outport(1),'DstPortHandle');
      | next_in = get_param(lh.Outport(1),'DstPortHandle');
      | 
      | %Delete connecting lines
      | delete_line(lh.Inport(1));
      | delete_line(lh.Outport(1));
      | delete_line(nb_lh.Outport(1));
      | 
      | % Generate new lines
      | add_line(gcb, last_out, next_in, 'autorouting', 'smart');
      | add_line(gcb, next_out, this_in, 'autorouting', 'smart');
      | add_line(gcb, this_out, next_but_one_in, 'autorouting', 'smart');
      | 
      | %Rearrange system
      | Simulink.BlockDiagram.arrangeSystem(gcb);
      | 
      | %Refresh
      | treeValues = FailureInjectionPointHelper.getAllFmAndParamsAsTreeString(gcb);
      | mo = Simulink.Mask.get(gcb);
      | dc = mo.getDialogControl('GbFmInfo');
      | treeView = dc.getDialogControl('TreeViewFM');
      | treeView.TreeItems = {};
      | treeView.TreeItems = treeValues;
      mask DialogControl TreeViewFM Prompt: Failure Mode Information
      mask DialogControl BtnOpen Prompt: Open FIP
      mask DialogControl BtnOpen Callback: open_system(gcb,'force');
      mask DialogControl BtnNew Prompt: New
      mask DialogControl BtnNew Callback:
      | dialog_fipManager_single(gcb, '');
      | 
      | %Enable move, edit, delete buttons
      | mo = Simulink.Mask.get(gcb);
      | mo.getDialogControl('BtnMoveUp').Enabled = 'on';
      | mo.getDialogControl('BtnMoveDown').Enabled = 'on';
      | mo.getDialogControl('BtnEdit').Enabled = 'on';
      | mo.getDialogControl('BtnDelete').Enabled = 'on';
      mask DialogControl BtnEdit Prompt: Edit
      mask DialogControl BtnEdit Callback:
      | mo = Simulink.Mask.get(gcb);
      | dc = mo.getDialogControl('GbFmInfo');
      | treeView = dc.getDialogControl('TreeViewFM');
      | try
      |     a = treeView.getSelectedItems();
      |     p = split(a, '/');
      | catch
      |     return;
      | end
      | dialog_fipManager_single(gcb, p{1});
      mask DialogControl BtnDelete Prompt: Delete
      mask DialogControl BtnDelete Callback:
      | %Get name of the failure mode block
      | mo = Simulink.Mask.get(gcb);
      | dc = mo.getDialogControl('GbFmInfo');
      | treeView = dc.getDialogControl('TreeViewFM');
      | try
      |     a = treeView.getSelectedItems();
      |     p = split(a, '/'); %name of failure mode block is p{1}
      | catch
      |     return;
      | end
      | 
      | %Save outport handle of the last and inport handle of the next block
      | lh = get_param([gcb,'/',p{1}],'LineHandles');
      | last_out = get_param(lh.Inport(1),'SrcPortHandle');
      | next_in = get_param(lh.Outport(1),'DstPortHandle');
      | 
      | %Delete connecting lines and failure mode block
      | delete_line(lh.Inport(1));
      | delete_line(lh.Outport(1));
      | fm_handle = get_param([gcb,'/',p{1}],'Handle');
      | delete_block(fm_handle);
      | 
      | % Generate new line from outport last to inport next
      | add_line(gcb, last_out, next_in, 'autorouting', 'smart');
      | 
      | %Rearrange system
      | Simulink.BlockDiagram.arrangeSystem(gcb);
      | 
      | %Disable move, edit, delete buttons in case all FMs are deleted
      | last_block = get_param(last_out,'Parent');
      | last_is_inport = strcmp(get_param(last_block,'BlockType'),'Inport');
      | next_block = get_param(next_in,'Parent');
      | next_is_outport = strcmp(get_param(next_block,'BlockType'),'Outport');
      | if (last_is_inport && next_is_outport)
      |     mo.getDialogControl('BtnMoveUp').Enabled = 'off';
      |     mo.getDialogControl('BtnMoveDown').Enabled = 'off';
      |     mo.getDialogControl('BtnEdit').Enabled = 'off';
      |     mo.getDialogControl('BtnDelete').Enabled = 'off';
      | end
      | 
      | %Refresh
      | treeValues = FailureInjectionPointHelper.getAllFmAndParamsAsTreeString(gcb);
      | mo = Simulink.Mask.get(gcb);
      | dc = mo.getDialogControl('GbFmInfo');
      | treeView = dc.getDialogControl('TreeViewFM');
      | treeView.TreeItems = {};
      | treeView.TreeItems = treeValues;
      mask DialogControl BtnRefresh Prompt: Refresh
      mask DialogControl BtnRefresh Callback:
      | set_param(gcb,'LinkStatus','none');
      | 
      | treeValues = FailureInjectionPointHelper.getAllFmAndParamsAsTreeString(gcb);
      | mo = Simulink.Mask.get(gcb);
      | dc = mo.getDialogControl('GbFmInfo');
      | treeView = dc.getDialogControl('TreeViewFM');
      | treeView.TreeItems = {};
      | treeView.TreeItems = treeValues;
      mask Display: image('icons/failure_injection_point.png','center')
  Out1 : Outport
  wires:
  In1/1 -> Handle sensor FIP1/1(In1)
  Handle sensor FIP1/1(Out1) -> Out1/1
